simulink model "DF_preview_pid_control"  (R2020b)
settings: Solver=VariableStepAuto  StartTime=0.01  StopTime=15  RelTol=1e-3
undefined symbols (not defined in the file): aubr, tablebr, vubr
libraries: pid_lib x2, Solver_SF x1, simulink x1
settings Model: Creator=wwcong  LastModifiedBy=85304
settings DataIOCC: ReturnWorkspaceOutputs=off
settings DebuggingCC: ArithmeticOperatorsInVariantConditions=warning
settings SFSimCC: SimUseLocalCustomCode=off  CustomCodeUndefinedFunction=UseInterfaceOnly
settings RTWCC: RTWUseLocalCustomCode=off

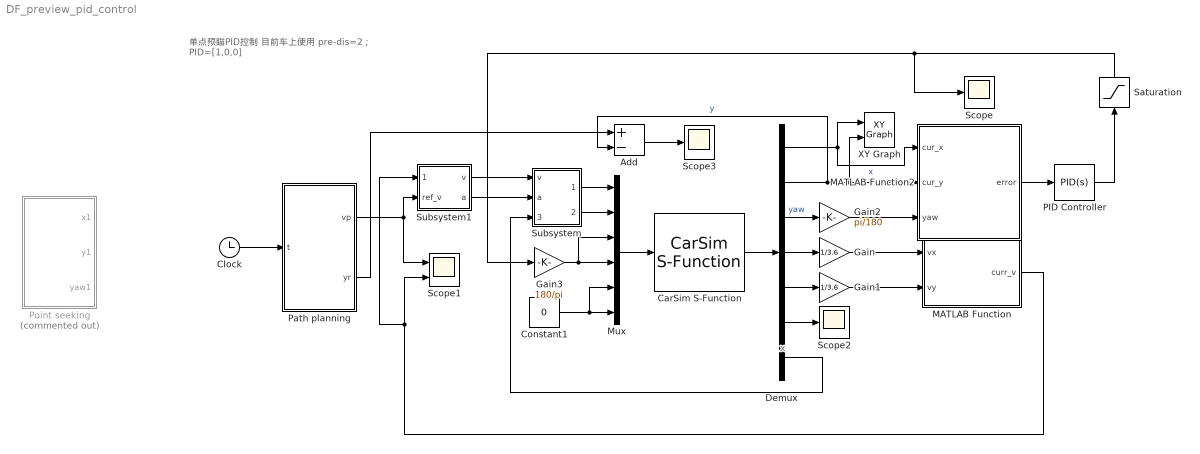
== system DF_preview_pid_control ==
  note: 单点预瞄PID控制
      | 目前车上使用
      | pre-dis=2；
      | PID=[1,0,0]
  note: x
  Add : Sum  Inputs=+-
  CarSim S-Function : Solver_SF/CarSim S-Function  Priority=1  SIMFILE=Radar_Acc_ExtSen_Car_1.sim
  Clock : Clock
  Constant1 : Constant  Value=0
  Demux : Demux  Outputs=7
  Gain : Gain  Gain=1/3.6
  Gain1 : Gain  Gain=1/3.6
  Gain2 : Gain  Gain=pi/180
  Gain3 : Gain  Gain=180/pi
  MATLAB Function : MATLAB Function  TreatAsAtomicUnit=on
  MATLAB Function2 : MATLAB Function  TreatAsAtomicUnit=on
  Mux : Mux  Inputs=6
  PID Controller : pid_lib/PID Controller  Controller=PID  Form=Parallel  TimeDomain=Continuous-time  UseExternalTs=off  SampleTime=-1  IntegratorMethod=Forward Euler  FilterMethod=Forward Euler  ControllerParametersSource=internal  P=1  I=0  D=0  UseFilter=on  N=100  TunerSelectOption=Transfer Function Based (PID Tuner App)  InitialConditionSource=internal  InitialConditionForIntegrator=0  InitialConditionForFilter=0  DifferentiatorICPrevScaledInput=0  ExternalReset=none  TrackingMode=off  Kt=1  LimitOutput=off  SatLimitsSource=internal  UpperSaturationLimit=inf  LowerSaturationLimit=-inf  LinearizeAsGain=on  AntiWindupMode=none  Kb=1  POutMin=[]  POutMax=[]  IOutMin=[]  IOutMax=[]  DOutMin=[]  DOutMax=[]  NOutMin=[]  NOutMax=[]  SumOutMin=[]  SumOutMax=[]  SaturationOutMin=[]  SaturationOutMax=[]  PParamMin=[]  PParamMax=[]  IParamMin=[]  IParamMax=[]  DParamMin=[]  DParamMax=[]  NParamMin=[]  NParamMax=[]  KbParamMin=[]  KbParamMax=[]  KtParamMin=[]  KtParamMax=[]  KbOutMin=[]  KbOutMax=[]  KtOutMin=[]  KtOutMax=[]  IntegratorOutMin=[]  IntegratorOutMax=[]  FilterOutMin=[]  FilterOutMax=[]  SumI1OutMin=[]  SumI1OutMax=[]  SumI2OutMin=[]  SumI2OutMax=[]  SumI3OutMin=[]  SumI3OutMax=[]  SumI4OutMin=[]  SumI4OutMax=[]  SumDOutMin=[]  SumDOutMax=[]  DifferentiatorOutMin=[]  DifferentiatorOutMax=[]  FilterDiffOutCoefMin=[]  FilterDiffOutCoefMax=[]  ReciprocalOutMin=[]  ReciprocalOutMax=[]  SumDenOutMin=[]  SumDenOutMax=[]  SumNumOutMin=[]  SumNumOutMax=[]  DivideOutMin=[]  DivideOutMax=[]  UdiffTsProdOutMin=[]  UdiffTsProdOutMax=[]  NTsProdOutMin=[]  NTsProdOutMax=[]  UintegralTsProdOutMin=[]  UintegralTsProdOutMax=[]  UngainTsProdOutMin=[]  UngainTsProdOutMax=[]  IntegratorContinuousStateAttributes=''  IntegratorStateMustResolveToSignalObject=off  IntegratorRTWStateStorageClass=Auto  FilterContinuousStateAttributes=''  FilterStateMustResolveToSignalObject=off  FilterRTWStateStorageClass=Auto  ParallelPVariant=InternalParameters  IdealPVariant=Disabled  IVariant=InternalParameters  DVariant=InternalParameters  IntegratorVariant=Continuous  SatVariant=Disabled  AWVariant=Passthrough  PCopyVariant=Disabled  TRVariant=Disabled  FdbkBlocksVariant=Forward  IdealPFdbkVariant=Disabled  SatFdbkVariant=Disabled  DerivativeFilterVariant=ContFilter  NVariant=InternalParameters  NCopyVariant=Disabled  FilterICVariant=InternalICsFilter  IntegratorICVariant=InternalICs  ExternalResetVariant=Disabled  TRSumVariant=Passthrough  SumFdbkVariant=Disabled  SumVariant=Sum_PID  TsampFilterVariant=InternalTs  TsampNgainVariant=Passthrough  TsampIntegralVariant=Passthrough  ExternalSaturationOutDataTypeStr=Inherit: Same as second input
  Path planning : MATLAB Function  TreatAsAtomicUnit=on
  Point seeking : MATLAB Function  Commented=on  TreatAsAtomicUnit=on
  Saturation : Saturate  UpperLimit=1  LowerLimit=-1
  Scope : Scope
  Scope1 : Scope  NumInputPorts=2
  Scope2 : Scope
  Scope3 : Scope
  Subsystem : Subsystem
  Subsystem1 : Subsystem
  XY Graph : simulink/Sinks/XY Graph  xmin=-10  xmax=60  ymin=-5  ymax=15  st=-1
  wires:
  CarSim S-Function/1 -> Demux/1
  Mux/1 -> CarSim S-Function/1
  Subsystem/1(torque) -> Mux/1
  Subsystem/2(brake) -> Mux/2
  Subsystem1/1(v) -> Subsystem/1(v)
  Demux/4 -> Gain/1
  Demux/5 -> Gain1/1
  Demux/7 -> Subsystem/3(rpm)
  Gain/1 -> MATLAB Function/1(vx)
  Gain1/1 -> MATLAB Function/2(vy)
  Clock/1 -> Path planning/1(t)
  Demux/3 -> Gain2/1  "yaw"
  Constant1/1 -> Mux/5, Mux/6
  Gain3/1 -> Mux/4, Mux/3
  Path planning/1(vp) -> Scope1/1, Subsystem1/2(ref_v)
  Subsystem1/2(a) -> Subsystem/2(a)
  Gain2/1 -> MATLAB Function2/3(yaw)
  Demux/1 -> XY Graph/1, MATLAB Function2/1(cur_x)  "x"
  Demux/2 -> MATLAB Function2/2(cur_y), XY Graph/2, Add/2  "y"
  MATLAB Function2/1(error) -> PID Controller/1
  PID Controller/1 -> Saturation/1
  Saturation/1 -> Scope/1, Gain3/1
  MATLAB Function/1(curr_v) -> Scope1/2, Subsystem1/1(current_v)
  Demux/6 -> Scope2/1
  Path planning/2(yr) -> Add/1
  Add/1 -> Scope3/1

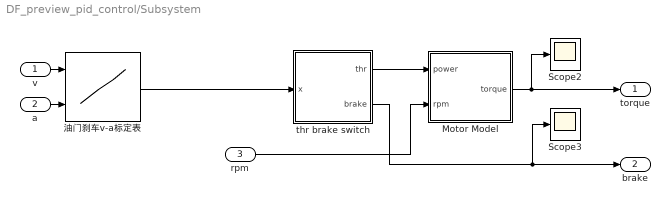
== system DF_preview_pid_control/Subsystem ==
  v : Inport
  a : Inport  Port=2
  rpm : Inport  Port=3
  Motor Model : MATLAB Function  TreatAsAtomicUnit=on
  Scope2 : Scope
  Scope3 : Scope
  thr brake switch : MATLAB Function  TreatAsAtomicUnit=on
  油门刹车v-a标定表 : Lookup_n-D  BreakpointsForDimension1=vubr  BreakpointsForDimension2=aubr  Table=tablebr  InternalRulePriority=Speed  RndMeth=Simplest  InputSameDT=on
      settings: InputPortMap=u0,u1
  torque : Outport
  brake : Outport  Port=2
  wires:
  v/1 -> 油门刹车v-a标定表/1
  thr brake switch/2(brake) -> brake/1, Scope3/1
  rpm/1 -> Motor Model/2(rpm)
  thr brake switch/1(thr) -> Motor Model/1(power)
  a/1 -> 油门刹车v-a标定表/2
  Motor Model/1(torque) -> torque/1, Scope2/1
  油门刹车v-a标定表/1 -> thr brake switch/1(x)

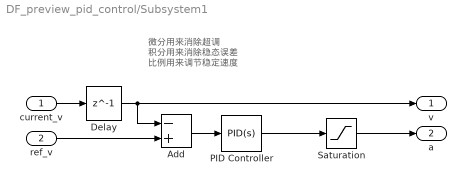
== system DF_preview_pid_control/Subsystem1 ==
  note: 微分用来消除超调
      | 积分用来消除稳态误差
      | 比例用来调节稳定速度
  current_v : Inport
  ref_v : Inport  Port=2
  Add : Sum  Inputs=-+
  Delay : Delay  DelayLength=1
  PID Controller : pid_lib/PID Controller  Controller=PID  Form=Parallel  TimeDomain=Continuous-time  UseExternalTs=off  SampleTime=-1  IntegratorMethod=Forward Euler  FilterMethod=Forward Euler  ControllerParametersSource=internal  P=8  I=0.1  D=0.1  UseFilter=on  N=30  TunerSelectOption=Transfer Function Based (PID Tuner App)  InitialConditionSource=internal  InitialConditionForIntegrator=0  InitialConditionForFilter=0  DifferentiatorICPrevScaledInput=0  ExternalReset=none  TrackingMode=off  Kt=1  LimitOutput=off  SatLimitsSource=internal  UpperSaturationLimit=inf  LowerSaturationLimit=-inf  LinearizeAsGain=on  AntiWindupMode=none  Kb=1  POutMin=[]  POutMax=[]  IOutMin=[]  IOutMax=[]  DOutMin=[]  DOutMax=[]  NOutMin=[]  NOutMax=[]  SumOutMin=[]  SumOutMax=[]  SaturationOutMin=[]  SaturationOutMax=[]  PParamMin=[]  PParamMax=[]  IParamMin=[]  IParamMax=[]  DParamMin=[]  DParamMax=[]  NParamMin=[]  NParamMax=[]  KbParamMin=[]  KbParamMax=[]  KtParamMin=[]  KtParamMax=[]  KbOutMin=[]  KbOutMax=[]  KtOutMin=[]  KtOutMax=[]  IntegratorOutMin=[]  IntegratorOutMax=[]  FilterOutMin=[]  FilterOutMax=[]  SumI1OutMin=[]  SumI1OutMax=[]  SumI2OutMin=[]  SumI2OutMax=[]  SumI3OutMin=[]  SumI3OutMax=[]  SumI4OutMin=[]  SumI4OutMax=[]  SumDOutMin=[]  SumDOutMax=[]  DifferentiatorOutMin=[]  DifferentiatorOutMax=[]  FilterDiffOutCoefMin=[]  FilterDiffOutCoefMax=[]  ReciprocalOutMin=[]  ReciprocalOutMax=[]  SumDenOutMin=[]  SumDenOutMax=[]  SumNumOutMin=[]  SumNumOutMax=[]  DivideOutMin=[]  DivideOutMax=[]  UdiffTsProdOutMin=[]  UdiffTsProdOutMax=[]  NTsProdOutMin=[]  NTsProdOutMax=[]  UintegralTsProdOutMin=[]  UintegralTsProdOutMax=[]  UngainTsProdOutMin=[]  UngainTsProdOutMax=[]  IntegratorContinuousStateAttributes=''  IntegratorStateMustResolveToSignalObject=off  IntegratorRTWStateStorageClass=Auto  FilterContinuousStateAttributes=''  FilterStateMustResolveToSignalObject=off  FilterRTWStateStorageClass=Auto  ParallelPVariant=InternalParameters  IdealPVariant=Disabled  IVariant=InternalParameters  DVariant=InternalParameters  IntegratorVariant=Continuous  SatVariant=Disabled  AWVariant=Passthrough  PCopyVariant=Disabled  TRVariant=Disabled  FdbkBlocksVariant=Forward  IdealPFdbkVariant=Disabled  SatFdbkVariant=Disabled  DerivativeFilterVariant=ContFilter  NVariant=InternalParameters  NCopyVariant=Disabled  FilterICVariant=InternalICsFilter  IntegratorICVariant=InternalICs  ExternalResetVariant=Disabled  TRSumVariant=Passthrough  SumFdbkVariant=Disabled  SumVariant=Sum_PID  TsampFilterVariant=InternalTs  TsampNgainVariant=Passthrough  TsampIntegralVariant=Passthrough  ExternalSaturationOutDataTypeStr=Inherit: Same as second input
  Saturation : Saturate  UpperLimit=5  LowerLimit=-8
  v : Outport
  a : Outport  Port=2
  wires:
  Delay/1 -> v/1, Add/1
  Add/1 -> PID Controller/1
  PID Controller/1 -> Saturation/1
  Saturation/1 -> a/1
  current_v/1 -> Delay/1
  ref_v/1 -> Add/2

== matlab function DF_preview_pid_control/Subsystem/thr brake switch ==
  data: x input; thr output; brake output
function [thr,brake] = trans(x)

    if(x>0)
        thr=x;
        brake=0;
    else 
        thr=0;
        brake=-x;
    end
end

== matlab function DF_preview_pid_control/Subsystem/Motor Model ==
  data: power input; torque output; rpm input
function torque = fcn(power,rpm)
Tmax=400*power;
    if(rpm<=4523)
        torque=Tmax;
    else 
        torque=Tmax*4523/rpm;
    end
end

== matlab function DF_preview_pid_control/MATLAB Function ==
  data: vx input; curr_v output; vy input
function curr_v = fcn(vx,vy)
curr_v=sqrt(vx^2+vy^2);

== matlab function DF_preview_pid_control/Point seeking ==
  data: x1 output; y1 output; yaw1 output
function [x1,y1,yaw1] = ref_path()
xo=50;
yo=5;
A=[1   0   0   0   0   0;                       % 求解五次多项式系数
   0   1   0   0   0   0;
   0   0   2   0   0   0;
   1   xo  xo^2  xo^3 xo^4  xo^5;
   0   1  2*xo 3*xo^2 4*xo^3 5*xo^4;
   0   0   2   6*xo 12*xo^2 20*xo^3];
B=[0;0;0;yo;0;0];
X5=linsolve(A,B);
x1=0:0.01:xo;
y1=X5(1)+X5(2).*x1+X5(3)*x1.^2+X5(4)*x1.^3+X5(5).*x1.^4+X5(6).*x1.^5;
y11=X5(2)+2*X5(3)*x1+3*X5(4)*x1.^2+4*X5(5).*x1.^3+5*X5(6).*x1.^4;
yaw1=atan(y11);

== matlab function DF_preview_pid_control/Path planning ==
  data: t input; vp output; yr output
%  function [vp,ap,xr,yr,thetar,kr] = fcn(t)
function [vp ,yr] = fcn(t)
    dx=50;
    dy=5;
    T=8;
    xstart=[0,0,0];
    xend=[dx,0,0];
    ystart=[0,0,0];
    yend=[dy,0,0];
    a=zeros(1,6);
    b=zeros(1,6);
    
    a(1)=xstart(1);
    a(2)=xstart(2);
    a(3)=xstart(3)/2;
    A1=[T^3,T^4,T^5;
        3*T^2,4*T^3,5*T^4;
        6*T,12*T^2,20*T^3];
    B1=[xend(1)-a(1)-a(2)*T-a(3)*T^2;
        xend(2)-a(2)-2*a(3)*T;
        xend(3)-2*a(3)];
    xs=inv(A1)*B1;
    a(4)=xs(1);
    a(5)=xs(2);
    a(6)=xs(3);
    b(1)=ystart(1);
    b(2)=ystart(2);
    b(3)=ystart(3)/2;
    A2=[dx^3,dx^4,dx^5;
        3*dx^2,4*dx^3,5*dx^4;
        6*dx,12*dx^2,20*dx^3];
    B2=[yend(1)-b(1)-b(2)*dx-b(3)*dx^2;
        yend(2)-b(2)-2*b(3)*dx;
        yend(3)-2*b(3)];
    ys=inv(A2)*B2;
    b(4)=ys(1);
    b(5)=ys(2);
    b(6)=ys(3);
    xr=a(1)+a(2)*t+a(3)*t^2+a(4)*t^3+a(5)*t^4+a(6)*t^5;
    yr=b(1)+b(2)*xr+b(3)*xr^2+b(4)*xr^3+b(5)*xr^4+b(6)*xr^5;
    xr_dot=a(2)+2*a(3)*t+3*a(4)*t^2+4*a(5)*t^3+5*a(6)*t^4;
    yr_dx=b(2)+2*b(3)*xr+3*b(4)*xr^2+4*b(5)*xr^3+5*b(6)*xr^4;
    yr_dot=yr_dx*xr_dot;
    thetar=atan(yr_dx);
    xr_dot2=2*a(3)+6*a(4)*t+12*a(5)*t^2+20*a(6)*t^3;
    yr_dx2=2*b(3)+6*b(4)*xr+12*b(5)*xr^2+20*b(6)*xr^3;
    yr_dot2=yr_dx2*xr_dot^2+yr_dx*xr_dot2;
    kr=yr_dx2/((1+yr_dx^2)^1.5);
    vp=sqrt(xr_dot^2+yr_dot^2);
    if xr_dot2>=0
        ap=sqrt(xr_dot2^2+yr_dot2^2);
    else
        ap=-sqrt(xr_dot2^2+yr_dot2^2);
    end

== matlab function DF_preview_pid_control/MATLAB Function2 ==
  data: cur_x input; cur_y input; yaw input; error output
function error  = fcn(cur_x,cur_y,yaw)
xo=50;
yo=5;
A=[1   0   0   0   0   0;                       % 求解五次多项式系数
   0   1   0   0   0   0;
   0   0   2   0   0   0;
   1   xo  xo^2  xo^3 xo^4  xo^5;
   0   1  2*xo 3*xo^2 4*xo^3 5*xo^4;
   0   0   2   6*xo 12*xo^2 20*xo^3];
B=[0;0;0;yo;0;0];
X5=linsolve(A,B);
x1=0:0.01:xo;
y1=X5(1)+X5(2).*x1+X5(3)*x1.^2+X5(4)*x1.^3+X5(5).*x1.^4+X5(6).*x1.^5;
y11=X5(2)+2*X5(3)*x1+3*X5(4)*x1.^2+4*X5(5).*x1.^3+5*X5(6).*x1.^4;
yaw1=atan(y11);

%% 预瞄
% pre_time = 1; %预瞄时长
pre_length = 2;


%% 车辆状态赋值
x = single(cur_x);
y = single(cur_y);
heading = yaw;

%%
%计算预瞄后车辆位置
pre_pose = zeros(1,2);
pre_pose(1) = x + pre_length*cos(heading);
pre_pose(2) = y + pre_length*sin(heading);

%%
%在参考轨迹上找实际参考点
%1.先找参考轨迹上离预瞄点最近的点
trajref=[x1;y1;yaw1]';
n = length(x1);
distmin = 1e5;
index = 1;
for i = 1:(n - 1)
    dist = sqrt((pre_pose(2)-trajref(i, 2)).*(pre_pose(2)-trajref(i, 2)) ...
        +(pre_pose(1)-trajref(i, 1)).*(pre_pose(1)-trajref(i, 1)));  
    if dist < distmin
        distmin = dist;
        index = i;    %排序，最小值索引
    end
end

%2.判断实际参考点位置
if index > 1
    temp = index;
    if (trajref(temp-1,1) < pre_pose(1))&& (pre_pose(1)<= trajref(temp,1))
        index = temp - 1;
    else
        if (trajref(temp-1,2) < pre_pose(2))&& (pre_pose(2)<= trajref(temp,2))
            index = temp - 1;
        end
    end
end
index;
%3.再找实际参考点
p0 = pre_pose(1:2);
p1 = trajref(index, 1:3);
p2 = trajref(index + 1, 1:3);
tol = 0.001;
ref_pose = zeros(1,4);
if abs(p2(1) - p1(1)) < tol    % p1和p2直线为平行于y轴的直线
    x = p1(1);     %投影点x坐标为p1的x坐标
    y = p0(2);     %投影点y坐标为p0的y坐标
elseif abs(p2(2) - p1(2)) < tol    % p1和p2直线为平行于x轴的直线
    x = p0(1);     %投影点x坐标为p0的x坐标
    y = p1(2);     %投影点y坐标为p1的y坐标
else
    k1 = (p2(2) - p1(2)) / (p2(1) - p1(1)); %p1和p2的直线斜率
    k2 = -1 / k1;   %p0和投影点的直线斜率，两者垂直
    x = (p0(2) - p1(2) + k1 * p1(1) - k2 * p0(1)) / (k1 - k2);
    y = p0(2) + k2 * (x - p0(1));
end
ref_pose(1) = x;
ref_pose(2) = y;
dist1 = sqrt((p2(2)-p1(2)).*(p2(2)-p1(2))+(p2(1)-p1(1)).*(p2(1)-p1(1)));%p1到p2的距离  
dist2 = sqrt((p2(2)-ref_pose(2)).*(p2(2)-ref_pose(2))+(p2(1)-ref_pose(1)).*(p2(1)-ref_pose(1)));%投影点到p2的距离
ratio = dist2 ./ dist1;
ref_pose(3) = ratio .* p1(3) + (1 - ratio) .* p2(3); %参考航向角

%%
%计算横向位置偏差
dx = pre_pose(1) - ref_pose(1);
dy = pre_pose(2) - ref_pose(2);

error = -1*(dy * cos(ref_pose(3)) - dx * sin(ref_pose(3)));
